simulink model "mppt_buck_boost_converterPV"  (R2021a)
settings: Solver=FixedStepDiscrete  StartTime=0.0  StopTime=inf  FixedStep=1e-6  RelTol=1e-3
undefined symbols (not defined in the file or in its folder): sigbuilder_block
libraries: spsSeriesRLCBranchLib x4, spsCurrentMeasurementLib x1, spsDCVoltageSourceLib x1, spsDiodeLib x1, spsMeanLib x1, spsMosfetLib x1, spsPVArrayLib x1, spsPWMGeneratorDCDCLib x1, spsVoltageMeasurementLib x1, spspowerguiLib x1
settings Model: SimulationMode=accelerator  Creator=karan  LastModifiedBy=karan

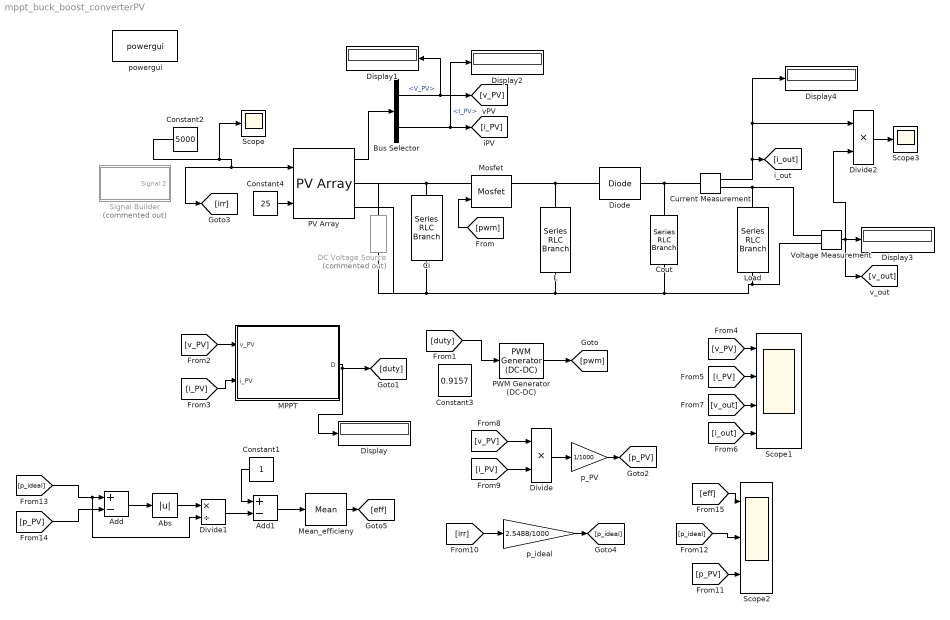
== system mppt_buck_boost_converterPV ==
  Abs : Abs
  Add : Sum  Inputs=+-
  Add1 : Sum  Inputs=+-
  Bus Selector : BusSelector  OutputSignals=V_PV,I_PV
  Ci : spsSeriesRLCBranchLib/Series RLC Branch  LConnTagsString=__new0  RConnTagsString=__new0  BranchType=RC  Resistance=1e-3  Inductance=1e-3  SetiL0=off  InitialCurrent=0  Capacitance=350e-6  Setx0=off  InitialVoltage=0  Measurements=None
  Constant1 : Constant
  Constant2 : Constant  Value=5000
  Constant3 : Constant  Value=0.9157
  Constant4 : Constant  Value=25
  Cout : spsSeriesRLCBranchLib/Series RLC Branch  LConnTagsString=__new0  RConnTagsString=__new0  BranchType=C  Resistance=1e-3  Inductance=1e-3  SetiL0=off  InitialCurrent=0  Capacitance=50e-6  Setx0=off  InitialVoltage=0  Measurements=None
  Current Measurement : spsCurrentMeasurementLib/Current Measurement  PhasorSimulation=off  OutputType=Complex  PSBequivalent=0
  DC Voltage Source : spsDCVoltageSourceLib/DC Voltage Source  Commented=on  Amplitude=160  Measurements=None
  Diode : spsDiodeLib/Diode  Ron=0.001  Lon=0  Vf=0.8  IC=0  UseSnubber=0  Rs=500  Cs=250e-9  Measurements=off
  Display{,1..4} (5 alike) : Display
  Divide : Product  Inputs=**
  Divide1 : Product  Inputs=*/
  Divide2 : Product  Inputs=**
  L : spsSeriesRLCBranchLib/Series RLC Branch  LConnTagsString=__new0  RConnTagsString=__new0  BranchType=L  Resistance=0.1  Inductance=4e-3  SetiL0=on  InitialCurrent=0  Capacitance=100e-6  Setx0=off  InitialVoltage=0  Measurements=Branch current
  Load : spsSeriesRLCBranchLib/Series RLC Branch  LConnTagsString=__new0  RConnTagsString=__new0  BranchType=R  Resistance=210  Inductance=1e-3  SetiL0=off  InitialCurrent=0  Capacitance=100e-6  Setx0=off  InitialVoltage=0  Measurements=None
  MPPT : MATLAB Function  TreatAsAtomicUnit=on
  Mean_efficieny : spsMeanLib/Mean  Freq=50  Vinit=0  Ts=1e-6
  Mosfet : spsMosfetLib/Mosfet  Ron=0.1  Lon=0  Rd=0.01  Vfd=0  IC=0  Rs=1e5  Cs=inf  Measurements=on
  PV Array : spsPVArrayLib/PV Array  Npar=2  Nser=5  PlotType=array @ 25 deg.C & specified irradiances  S_vec=[500 1000 1500 2000 2500 3000 3500 4000 4500 5000 5500 6000]  Temp_C_vec="[ 45 25  ]"  ModuleName=Vikram Solar Eldora VSP.60.255.03  PlotWhenSelected=off  Pm=254.888  Ncell=60  Voc=37.6  Isc=8.99  Vm=30.2  Im=8.44  beta_Voc_pc=-0.3426  alpha_Isc_pc=-0.012803  beta_Voc=-0.12882  alpha_Isc=-0.001151  IL=9.0196  I0=1.4661e-10  nI=0.98245  Rsh=267.647  Rs=0.34677  RobustModel=off  RobustCellTemperature=30  BAL=off  Tc=1e-6  Tfilter=1e-6
  PWM Generator (DC-DC) : spsPWMGeneratorDCDCLib/PWM Generator (DC-DC)  Fsw=25000  Ts=1e-6
  Scope : Scope
  Scope1 : Scope  NumInputPorts=4
  Scope2 : Scope  NumInputPorts=3
  Scope3 : Scope
  Signal Builder : Subsystem  Tag=STV Subsys  Commented=on  LoadFcn=sigbuilder_block('load');  StartFcn=sigbuilder_block('start');  StopFcn=sigbuilder_block('stop');  ClipboardFcn=sigbuilder_block('clipboard');  mask(Sigbuilder block){tuvar=[0:10]}
      mask help: Simulink:masks:SigbuilderBlock_MD
      mask init:
      | if ~strcmp(get_param(bdroot(gcbh),'SimulationStatus'),'stopped') tuvar = sigbuilder_block('maskInit'); end
      settings: CopyFcn=sigbuilder_block('copy');  DeleteFcn=sigbuilder_block('delete');  ModelCloseFcn=sigbuilder_block('modelClose');  PreSaveFcn=sigbuilder_block('preSave');  PauseFcn=sigbuilder_block('pause');  ContinueFcn=sigbuilder_block('continue');  NameChangeFcn=sigbuilder_block('namechange');  OpenFcn=sigbuilder_block('open',[14 176 550.5 254.5 ]);  CloseFcn=sigbuilder_block('close');
      mask Display: plot(0, 0, 100, 100,[2, 2, 32, 32, 2], [68, 8, 8, 68, 68],[32, 2], [38, 38], [32, 19, 2],[53, 60, 44], [32, 17, 17, 2],[16, 16, 31, 31]);txt = getActiveGroup(gcbh);text(2, 100, txt,'verticalAlignment', 'top');
  Voltage Measurement : spsVoltageMeasurementLib/Voltage Measurement  PhasorSimulation=off  OutputType=Complex  PSBequivalent=0
  p_PV : Gain  Gain=1/1000
  p_ideal : Gain  Gain=2.5488/1000
  powergui : spspowerguiLib/powergui  Priority=1  SimulationMode=Discrete  SampleTime=1e-6  frequency=60  Iterations=50  frequencyindice=0  Pbase=100e6  ErrMax=1e-4  UnitsV=kV  UnitsW=MW  buscounter=0  FunctionMessages=off  echomessages=off  EnableUseOfTLC=off  CurrentSourceSwitches=off  DisableSnubberDevices=off  DisableRonSwitches=off  DisableVfSwitches=off  DisplayEquations=off  AutomaticDiscreteSolvers=off  SolverType=Tustin/Backward Euler (TBE)  Interpol=off  ExternalGateDelay=off  methode=off  Ts=100  x0status=blocks  SPID=on  SwTol=0  HookPort=off  NonlinearTolerance=1e-4  nMaxIteration=100  ContinueOnMaxIteration=off  RestoreLinks=warning  ResistiveCurrentMeasurement=off  Frange=[0:2:500]  Ylog=off  Xlog=on  ShowGrid=off  save=off  variable=ZData  structure=0  ZoomFFT=off  StartTime=0.0  cycles=1  DisplayStyle=1  fundamental=60  FreqAxis=off  MaxFrequency=1000  frequencyindicesteady=1  RmsSteady=1  display=off
  wires:
  PV Array/1 -> Bus Selector/1
  Bus Selector/1 -> Display1/1, [v_PV]  "<V_PV>"
  Bus Selector/2 -> Display2/1, [i_PV]  "<I_PV>"
  Voltage Measurement/1 -> [v_out], Display3/1, Divide2/2
  Current Measurement/1 -> Display4/1, Divide2/1, [i_out]
  [pwm] -> Mosfet/1
  PWM Generator (DC-DC)/1 -> [pwm]
  [v_PV] -> MPPT/1(v_PV)
  [i_PV] -> MPPT/2(i_PV)
  MPPT/1(D) -> Display/1, [duty]
  [v_PV] -> Scope1/1
  [i_PV] -> Scope1/2
  [i_out] -> Scope1/4
  [v_out] -> Scope1/3
  [i_PV] -> Divide/2
  [v_PV] -> Divide/1
  Divide/1 -> p_PV/1
  p_PV/1 -> [p_PV]
  [irr] -> p_ideal/1
  p_ideal/1 -> [p_ideal]
  Add/1 -> Abs/1
  Abs/1 -> Divide1/1
  Constant1/1 -> Add1/1
  Divide1/1 -> Add1/2
  [p_ideal] -> Divide1/2, Add/1
  [p_PV] -> Add/2
  Add1/1 -> Mean_efficieny/1
  Mean_efficieny/1 -> [eff]
  [eff] -> Scope2/1
  Constant2/1 -> Scope/1, [irr], PV Array/1
  Constant4/1 -> PV Array/2
  Divide2/1 -> Scope3/1
  [p_PV] -> Scope2/3
  [p_ideal] -> Scope2/2
  [duty] -> PWM Generator (DC-DC)/1
  connections:
  Mosfet/LConn1 -- PV Array/RConn1 -- DC Voltage Source/RConn1 -- Ci/LConn1
  Voltage Measurement/LConn2 -- Load/RConn1 -- Cout/LConn1 -- L/RConn1 -- PV Array/RConn2 -- DC Voltage Source/LConn1 -- Ci/RConn1
  Cout/RConn1 -- Current Measurement/LConn1 -- Diode/LConn1
  Current Measurement/RConn1 -- Load/LConn1 -- Voltage Measurement/LConn1
  Mosfet/RConn1 -- Diode/RConn1 -- L/LConn1

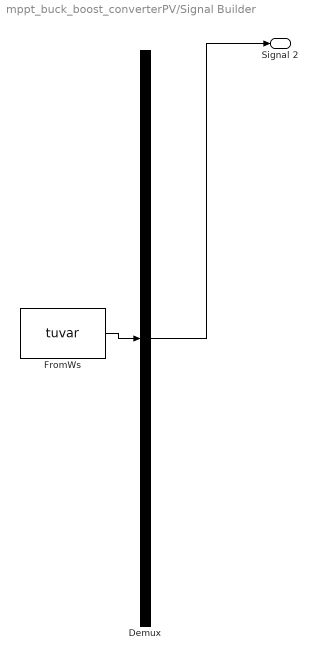
== system mppt_buck_boost_converterPV/Signal Builder ==
  Demux : Demux  Tag=STV Demux  Outputs=1
      settings: DisplayOption=none
  FromWs : FromWorkspace  Tag=STV FromWs  VariableName=tuvar
      SigBuilderData=|
      | common.afterFinalStr = 'Extrapolate'
      | common.sampleTime = 0
      | dataSet.timeRange = [0 40]
      | dataSet.name = 'Group 1'
      | sbobj.Groups.Name = 'Group 1'
      | sbobj.Groups.Signals.Name = 'Signal 2'
      | sbobj.Groups.Signals.XData = [0 0.109589041096 0.219178082192 0.328767123288 0.438356164384 0.547945205479 0.657534246575 0.767123287671 0.876712328767 0.986301369863 1.09589041096 1.20547945205 ... (366 elements, 1x366)]
      | sbobj.Groups.Signals.YData = [6.80381010226 6.81774386061 6.83268104702 6.84861398995 6.86553445948 6.88343366999 6.90230228315 6.92213041129 6.94290762101 6.96462293727 6.98726484776 7.01082130768 ... (366 elements, 1x366)]
      | sbobj.Groups.TimeRange = [0 40]
  Signal 2 : Outport  Tag=STV Outport
  wires:
  FromWs/1 -> Demux/1
  Demux/1 -> Signal 2/1

== matlab function mppt_buck_boost_converterPV/MPPT ==
  data: v_PV input; D output; i_PV input
function D  = mppt(v_PV,i_PV)

Dmax = 0.95;
Dmin = 0;
Dinit = 0.10;
deltaD = 0.01;

persistent vold pold Dold ;

dataType = 'double';

if isempty(vold)
    vold=0;
    pold=0;
    Dold=Dinit;
end

P = v_PV*i_PV;
dV = v_PV - vold;
dP = P - pold;

if(dP~=0)
    if(dP<0)
       if dV<0
           D = Dold - deltaD;
       else
           D = Dold + deltaD;
       end
    else
      if dV<0  
          D = Dold + deltaD;
      else
          D = Dold - deltaD;
      end
    end
else D= Dold;
end
          
if D>=Dmax || D<=Dmin
    D = Dold;
end

Dold= D;
vold = v_PV;
pold = P;

        



%persistent variable type can store the data
% we need the old data by obtaining difference 
%between old and new value
